simulink model "IO397_src"  (R2022b)
settings: Solver=FixedStepDiscrete  StartTime=0.0  StopTime=0.001  RelTol=1e-3
libraries: SG_library x1, hdlsllib x1
settings Model: DataTypeOverride=Off  Creator=mavolery  LastModifiedBy=mavolery
settings OptimizationCC: BlockReduction=off  ConditionallyExecuteInputs=off  DefaultParameterBehavior=Inlined  InheritOutputTypeSmallerThanSingle=on
settings DebuggingCC: AlgebraicLoopMsg=error  InheritedTsInSrcMsg=none  SingleTaskRateTransMsg=error
settings HardwareCC: ProdBitPerPointer=32  ProdBitPerSizeT=32  ProdBitPerPtrDiffT=32  ProdLargestAtomicFloat=None  ProdIntDivRoundTo=Undefined  ProdEndianess=Unspecified  ProdWordSize=32  ProdHWDeviceType=ASIC/FPGA->ASIC/FPGA  TargetBitPerPointer=64  TargetBitPerSizeT=64  TargetBitPerPtrDiffT=64  TargetLongLongMode=on  TargetIntDivRoundTo=Zero  TargetEndianess=LittleEndian  TargetWordSize=64  TargetHWDeviceType=Custom Processor->MATLAB Host Computer  ProdEqTarget=off

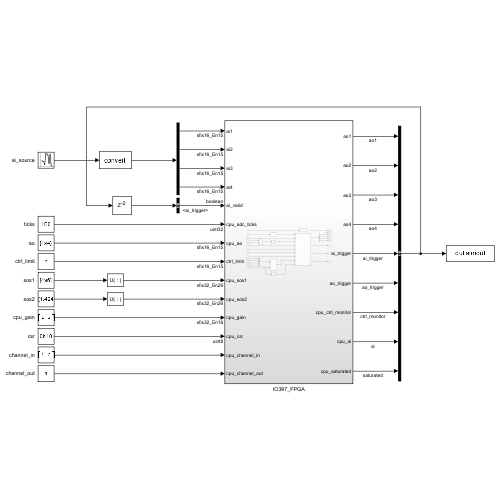
[thumbnail: Simulink's stored preview of the top-level diagram]
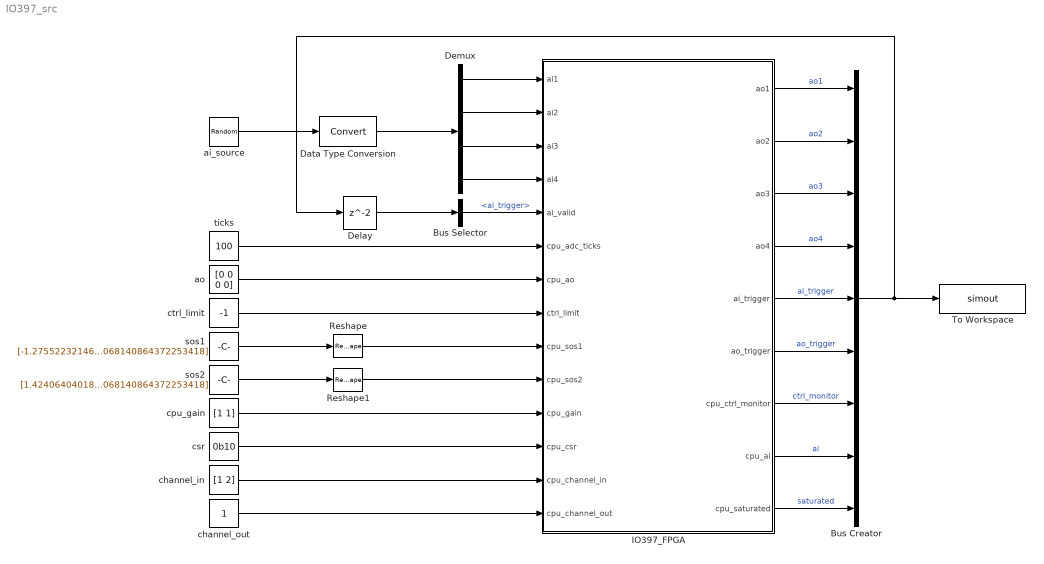
== system IO397_src ==
  Bus Creator : BusCreator  Inputs=9
  Bus Selector : BusSelector  OutputSignals=ai_trigger
  Data Type Conversion : DataTypeConversion  SaturateOnIntegerOverflow=off  RndMeth=Floor
  Delay : Delay
  Demux : Demux
  IO397_FPGA : Subsystem
  Reshape : Reshape
  Reshape1 : Reshape
  To Workspace : ToWorkspace  VariableName=simout  SaveFormat=Timeseries  SampleTime=-1
  ai_source : RandomNumber  Variance=1e-3  Seed=0:3
  ao : Constant  Value=[0 0 0 0]  OutDataTypeStr=Inherit: Inherit via back propagation  SampleTime=-1
  channel_in : Constant  Value=[1 2]  OutDataTypeStr=Inherit: Inherit via back propagation  SampleTime=-1
  channel_out : Constant  OutDataTypeStr=Inherit: Inherit via back propagation  SampleTime=-1
  cpu_gain : Constant  Value=[1 1]  OutDataTypeStr=Inherit: Inherit via back propagation  SampleTime=-1
  csr : Constant  Value=0b10  OutDataTypeStr=Inherit: Inherit via back propagation  SampleTime=-1
  ctrl_limit : Constant  Value=-1  OutDataTypeStr=Inherit: Inherit via back propagation  SampleTime=-1
  sos1 : Constant  Value=[-1.2755223214626312256 1.257218480110168457 2.0602753758430480957 1 -0.095409825444221496582 -0.067025259137153625488;3.0412670820951461792 -2.5177141278982162476 0.50291076302528381348 1 -0.89835710823535919189 0.20038597285747528076;0.096603438258171081543 0.030124843120574951172 0.0076837837696075439453 1 1.5939609259366989136 0.61575837433338165283;3.223117828369140625 3.0878312289714813232 1.4877308458089828491 1 0.98293107748031616211 0.46068140864372253418]  OutDataTypeStr=Inherit: Inherit via back propagation  SampleTime=-1
  sos2 : Constant  Value=[1.4240640401840209961 3.9948539882898330688 1.9990000426769256592 1 -0.095409825444221496582 -0.067025259137153625488;2.6892739087343215942 0.33791068196296691895 -0.35225719213485717773 1 -0.89835710823535919189 0.20038597285747528076;0.086499780416488647461 -0.085405886173248291016 0.021359235048294067383 1 1.5939609259366989136 0.61575837433338165283;8.7784139066934585571 8.6148883402347564697 4.0032984465360641479 1 0.98293107748031616211 0.46068140864372253418]  OutDataTypeStr=Inherit: Inherit via back propagation  SampleTime=-1
  ticks : Constant  Value=100  OutDataTypeStr=Inherit: Inherit via back propagation  SampleTime=-1
  wires:
  IO397_FPGA/6(ao_trigger) -> Bus Creator/6  "ao_trigger"
  IO397_FPGA/3(ao3) -> Bus Creator/3  "ao3"
  Reshape/1 -> IO397_FPGA/9(cpu_sos1)
  sos1/1 -> Reshape/1
  cpu_gain/1 -> IO397_FPGA/11(cpu_gain)
  ticks/1 -> IO397_FPGA/6(cpu_adc_ticks)
  IO397_FPGA/5(ai_trigger) -> Bus Creator/5  "ai_trigger"
  ao/1 -> IO397_FPGA/7(cpu_ao)
  IO397_FPGA/4(ao4) -> Bus Creator/4  "ao4"
  IO397_FPGA/2(ao2) -> Bus Creator/2  "ao2"
  IO397_FPGA/1(ao1) -> Bus Creator/1  "ao1"
  ctrl_limit/1 -> IO397_FPGA/8(ctrl_limit)
  csr/1 -> IO397_FPGA/12(cpu_csr)
  sos2/1 -> Reshape1/1
  IO397_FPGA/8(cpu_ai) -> Bus Creator/8  "ai"
  Bus Creator/1 -> Delay/1, To Workspace/1
  Reshape1/1 -> IO397_FPGA/10(cpu_sos2)
  IO397_FPGA/7(cpu_ctrl_monitor) -> Bus Creator/7  "ctrl_monitor"
  ai_source/1 -> Data Type Conversion/1
  Data Type Conversion/1 -> Demux/1
  Demux/1 -> IO397_FPGA/1(ai1)
  Demux/2 -> IO397_FPGA/2(ai2)
  Demux/3 -> IO397_FPGA/3(ai3)
  Demux/4 -> IO397_FPGA/4(ai4)
  Bus Selector/1 -> IO397_FPGA/5(ai_valid)  "<ai_trigger>"
  Delay/1 -> Bus Selector/1
  channel_in/1 -> IO397_FPGA/13(cpu_channel_in)
  channel_out/1 -> IO397_FPGA/14(cpu_channel_out)
  IO397_FPGA/9(cpu_saturated) -> Bus Creator/9  "saturated"

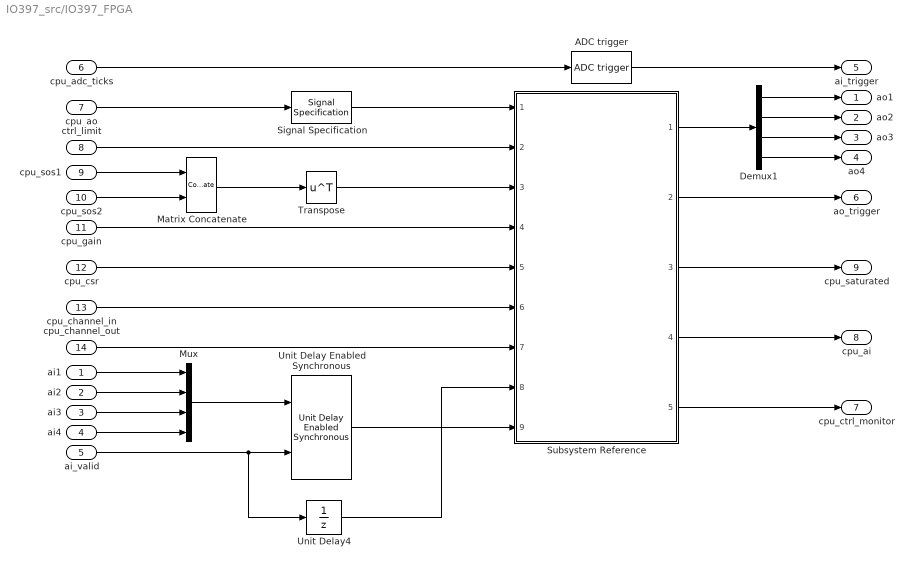
== system IO397_src/IO397_FPGA ==
  ai1 : Inport  OutDataTypeStr=fixdt(1,16,15)
  ai2 : Inport  Port=2  OutDataTypeStr=fixdt(1,16,15)
  ai3 : Inport  Port=3  OutDataTypeStr=fixdt(1,16,15)
  ai4 : Inport  Port=4  OutDataTypeStr=fixdt(1,16,15)
  ai_valid : Inport  Port=5  OutDataTypeStr=boolean
  cpu_adc_ticks : Inport  Port=6  OutDataTypeStr=uint32
  cpu_ao : Inport  Port=7  OutDataTypeStr=fixdt(1,16,15)
  ctrl_limit : Inport  Port=8  OutDataTypeStr=fixdt(1,16,15)
  cpu_sos1 : Inport  Port=9  OutDataTypeStr=fixdt(1,32,26)
  cpu_sos2 : Inport  Port=10  OutDataTypeStr=fixdt(1,32,26)
  cpu_gain : Inport  Port=11  OutDataTypeStr=fixdt(1,32,16)
  cpu_csr : Inport  Port=12  OutDataTypeStr=uint8
  cpu_channel_in : Inport  Port=13
  cpu_channel_out : Inport  Port=14
  ADC trigger : SG_library/Source elements/ADC trigger
      settings: SourceProductName=Custom Speedgoat implementations
  Demux1 : Demux
  Matrix Concatenate : Concatenate  Mode=Multidimensional array  ConcatenateDimension=2
  Mux : Mux
  Signal Specification : SignalSpecification  SampleTime=10e-9
  Subsystem Reference : Subsystem  ReferencedSubsystem=control_filter
  Transpose : Math  Operator=transpose
  Unit Delay Enabled Synchronous : hdlsllib/Discrete/Unit Delay Enabled Synchronous  InitialCondition=0.0  SampleTime=-1
  Unit Delay4 : UnitDelay  SampleTime=-1  HasFrameUpgradeWarning=on
  ao1 : Outport  VectorParamsAs1DForOutWhenUnconnected=off
  ao2 : Outport  Port=2  VectorParamsAs1DForOutWhenUnconnected=off
  ao3 : Outport  Port=3  VectorParamsAs1DForOutWhenUnconnected=off
  ao4 : Outport  Port=4  VectorParamsAs1DForOutWhenUnconnected=off
  ai_trigger : Outport  Port=5  VectorParamsAs1DForOutWhenUnconnected=off
  ao_trigger : Outport  Port=6  VectorParamsAs1DForOutWhenUnconnected=off
  cpu_ctrl_monitor : Outport  Port=7  VectorParamsAs1DForOutWhenUnconnected=off
  cpu_ai : Outport  Port=8  VectorParamsAs1DForOutWhenUnconnected=off
  cpu_saturated : Outport  Port=9
  wires:
  ai1/1 -> Mux/1
  ai2/1 -> Mux/2
  ai3/1 -> Mux/3
  ai4/1 -> Mux/4
  Mux/1 -> Unit Delay Enabled Synchronous/1
  Demux1/1 -> ao1/1
  Demux1/2 -> ao2/1
  Demux1/3 -> ao3/1
  Demux1/4 -> ao4/1
  ai_valid/1 -> Unit Delay Enabled Synchronous/2, Unit Delay4/1
  cpu_ao/1 -> Signal Specification/1
  ctrl_limit/1 -> Subsystem Reference/2
  cpu_gain/1 -> Subsystem Reference/4
  cpu_csr/1 -> Subsystem Reference/5
  ADC trigger/1 -> ai_trigger/1
  cpu_adc_ticks/1 -> ADC trigger/1
  cpu_sos1/1 -> Matrix Concatenate/1
  cpu_sos2/1 -> Matrix Concatenate/2
  Matrix Concatenate/1 -> Transpose/1
  Transpose/1 -> Subsystem Reference/3
  Signal Specification/1 -> Subsystem Reference/1
  Subsystem Reference/1 -> Demux1/1
  Subsystem Reference/2 -> ao_trigger/1
  Subsystem Reference/3 -> cpu_saturated/1
  Subsystem Reference/4 -> cpu_ai/1
  cpu_channel_in/1 -> Subsystem Reference/6
  cpu_channel_out/1 -> Subsystem Reference/7
  Unit Delay4/1 -> Subsystem Reference/8
  Unit Delay Enabled Synchronous/1 -> Subsystem Reference/9
  Subsystem Reference/5 -> cpu_ctrl_monitor/1
